simulink model "SistemaGrua_ModeloPlanta"  (R2020b)
settings: Solver=VariableStepAuto  StartTime=0.0  StopTime=10  RelTol=1e-3
values from neighbouring files (symbols this model uses):
  bhb = 1e8    (= 100000000)    [Valores.m]    (also in Valores_1.m; valoresPlanta.m; valoresPlanta_29_9_24.m; valoresPlanta_V3.m)
  bhEb = 2.2e9    (= 2200000000)    [Valores.m]    (also in Valores_1.m; valoresPlanta.m; valoresPlanta_29_9_24.m; valoresPlanta_V3.m)
  bhm = 18    [Valores.m]    (also in Valores_1.m; valoresPlanta.m; valoresPlanta_29_9_24.m; valoresPlanta_V3.m)
  bwu = 150    [Valores.m]    (also in Valores_1.m; valoresPlanta.m; valoresPlanta_29_9_24.m; valoresPlanta_V3.m)
  ih = 22    [Valores.m]    (also in Valores_1.m; valoresPlanta.m; valoresPlanta_29_9_24.m; valoresPlanta_V3.m)
  it = 30    [Valores.m]    (also in Valores_1.m; valoresPlanta.m; valoresPlanta_29_9_24.m; valoresPlanta_V3.m)
  Jhm_hb = 30    [Valores.m]    (also in Valores_1.m; valoresPlanta.m; valoresPlanta_29_9_24.m; valoresPlanta_V3.m)
  kwu = 2.36e8    (= 236000000)    [Valores.m]    (also in Valores_1.m; valoresPlanta.m; valoresPlanta_29_9_24.m; valoresPlanta_V3.m)
  rhd = 0.75    [Valores.m]    (also in Valores_1.m; valoresPlanta.m; valoresPlanta_29_9_24.m; valoresPlanta_V3.m)
  rtd = 0.5    [Valores.m]    (also in Valores_1.m; valoresPlanta.m; valoresPlanta_29_9_24.m; valoresPlanta_V3.m)
  tauhm = 1e-3    (= 0.001)    [Valores.m]    (also in Valores_1.m)
  Thb_Max = 5e4    (= 50000)    [Valores.m]    (also in Valores_1.m; valoresPlanta.m; valoresPlanta_29_9_24.m; valoresPlanta_V3.m)
  ThEb_Max = 1.1e6    (= 1100000)    [Valores.m]    (also in Valores_1.m; valoresPlanta.m; valoresPlanta_29_9_24.m; valoresPlanta_V3.m)
  Yt0 = 45    [Valores.m]    (also in Valores_1.m; valoresPlanta.m; valoresPlanta_29_9_24.m; valoresPlanta_V3.m)
undefined symbols (not defined in the file or in its folder): beqc, Meqc, sigbuilder_block
settings Model: Creator=Matias  LastModifiedBy=agustin

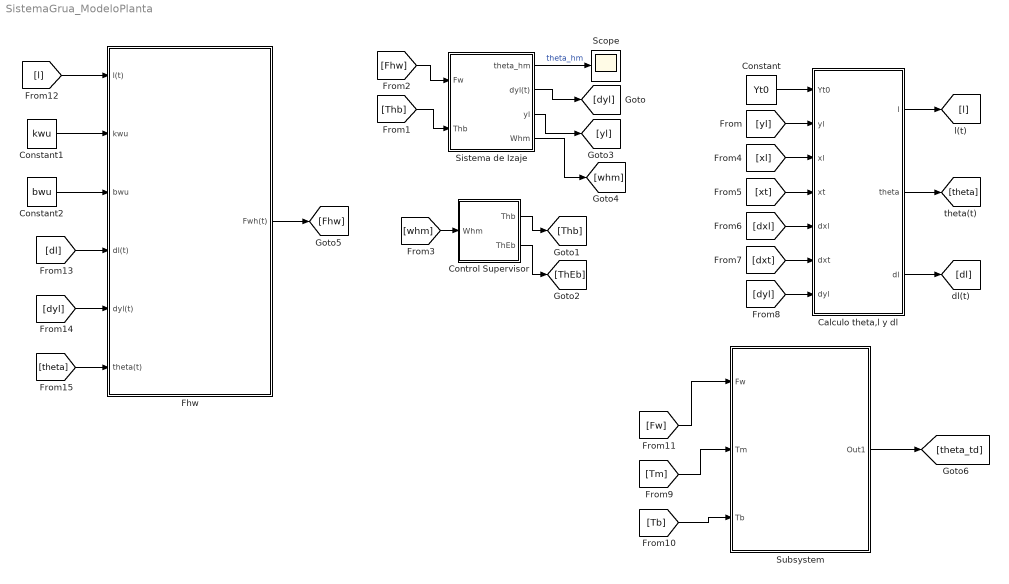
== system SistemaGrua_ModeloPlanta ==
  Calculo theta,l y dl : Subsystem
  Constant : Constant  Value=Yt0
  Constant1 : Constant  Value=kwu
  Constant2 : Constant  Value=bwu
  Control Supervisor : Subsystem
  Fhw : Subsystem
  Scope : Scope
  Sistema de Izaje : Subsystem
  Subsystem : Subsystem
  wires:
  [whm] -> Control Supervisor/1(Whm)
  Control Supervisor/1(Thb) -> [Thb]
  Sistema de Izaje/2(dyl(t)) -> [dyl]
  [Thb] -> Sistema de Izaje/2(Thb)
  [Fhw] -> Sistema de Izaje/1(Fw)
  Control Supervisor/2(ThEb) -> [ThEb]
  Sistema de Izaje/1(theta_hm) -> Scope/1  "theta_hm"
  Calculo theta,l y dl/1(l) -> [l]
  Calculo theta,l y dl/2(theta) -> [theta]
  Constant/1 -> Calculo theta,l y dl/1(Yt0)
  [xt] -> Calculo theta,l y dl/4(xt)
  [xl] -> Calculo theta,l y dl/3(xl)
  [yl] -> Calculo theta,l y dl/2(yl)
  Calculo theta,l y dl/3(dl) -> [dl]
  [dyl] -> Calculo theta,l y dl/7(dyl)
  [dxt] -> Calculo theta,l y dl/6(dxt)
  [dxl] -> Calculo theta,l y dl/5(dxl)
  Fhw/1(Fwh(t)) -> [Fhw]
  [theta] -> Fhw/6(theta(t))
  [dyl] -> Fhw/5(dyl(t))
  [dl] -> Fhw/4(dl(t))
  [l] -> Fhw/1(l(t))
  Constant1/1 -> Fhw/2(kwu)
  Constant2/1 -> Fhw/3(bwu)
  Sistema de Izaje/3(yl) -> [yl]
  Sistema de Izaje/4(Whm) -> [whm]
  [Tb] -> Subsystem/3(Tb)
  [Fw] -> Subsystem/1(Fw)
  [Tm] -> Subsystem/2(Tm)
  Subsystem/1(Out1) -> [theta_td]

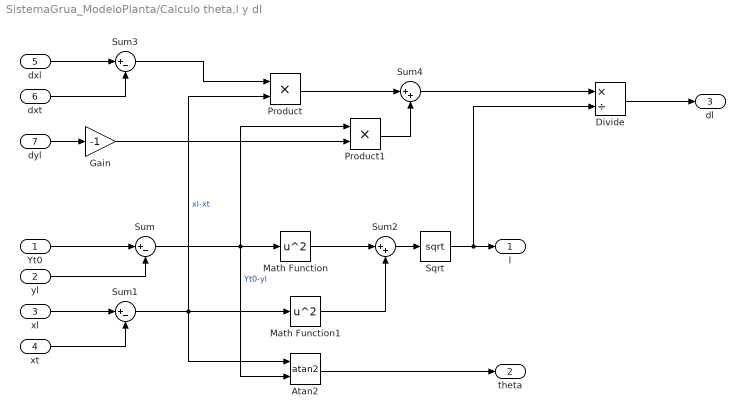
== system SistemaGrua_ModeloPlanta/Calculo theta,l y dl ==
  Yt0 : Inport
  yl : Inport  Port=2
  xl : Inport  Port=3
  xt : Inport  Port=4
  dxl : Inport  Port=5
  dxt : Inport  Port=6
  dyl : Inport  Port=7
  Atan2 : Trigonometry  Operator=atan2
  Divide : Product  Inputs=*/
  Gain : Gain  Gain=-1
  Math Function : Math  Operator=square  SaturateOnIntegerOverflow=on
  Math Function1 : Math  Operator=square  SaturateOnIntegerOverflow=on
  Product : Product
  Product1 : Product
  Sqrt : Sqrt  SaturateOnIntegerOverflow=on
  Sum : Sum  Inputs=|+-
  Sum1 : Sum  Inputs=|+-
  Sum2 : Sum  Inputs=|++
  Sum3 : Sum  Inputs=|+-
  Sum4 : Sum  Inputs=|++
  l : Outport
  theta : Outport  Port=2
  dl : Outport  Port=3
  wires:
  Yt0/1 -> Sum/1
  yl/1 -> Sum/2
  xl/1 -> Sum1/1
  xt/1 -> Sum1/2
  Atan2/1 -> theta/1
  Sum1/1 -> Product/2, Math Function1/1, Atan2/1  "xl-xt"
  Sum/1 -> Product1/1, Atan2/2, Math Function/1  "Yt0-yl"
  Math Function/1 -> Sum2/1
  Math Function1/1 -> Sum2/2
  Sum2/1 -> Sqrt/1
  Sqrt/1 -> Divide/2, l/1
  dxl/1 -> Sum3/1
  dxt/1 -> Sum3/2
  Sum3/1 -> Product/1
  dyl/1 -> Gain/1
  Gain/1 -> Product1/2
  Product/1 -> Sum4/1
  Product1/1 -> Sum4/2
  Sum4/1 -> Divide/1
  Divide/1 -> dl/1

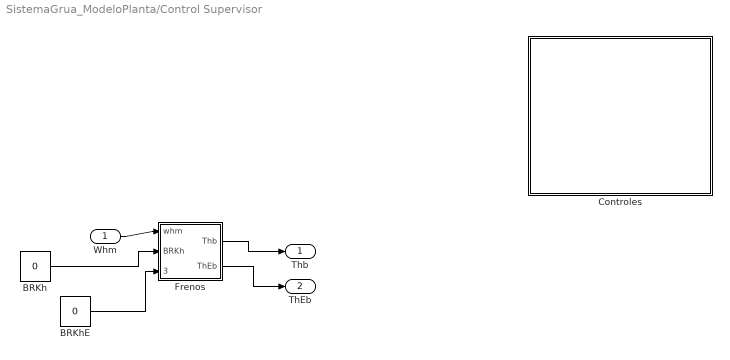
== system SistemaGrua_ModeloPlanta/Control Supervisor ==
  Whm : Inport
  BRKh : Constant  Value=0
  BRKhE : Constant  Value=0
  Controles : Subsystem
  "Frenos " : Stateflow chart  TreatAsAtomicUnit=on
  Thb : Outport
  ThEb : Outport  Port=2
  wires:
  "Frenos "/1(Thb) -> Thb/1
  BRKh/1 -> "Frenos "/2(BRKh)
  Whm/1 -> "Frenos "/1(whm)
  BRKhE/1 -> "Frenos "/3(BRKhE)
  "Frenos "/2(ThEb) -> ThEb/1

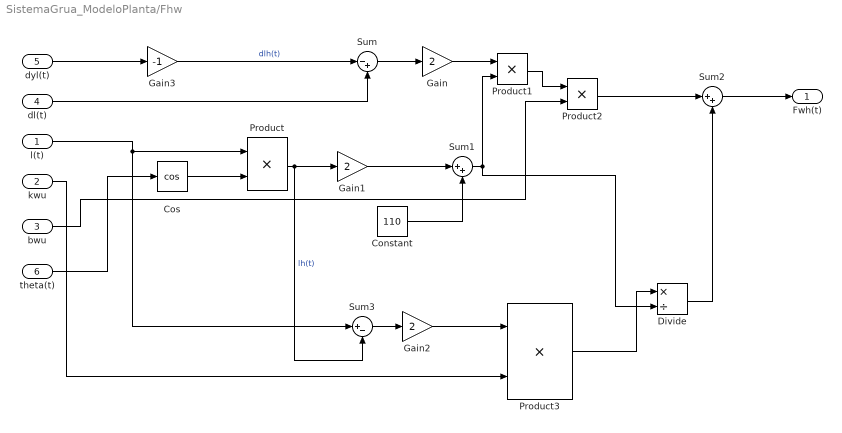
== system SistemaGrua_ModeloPlanta/Fhw ==
  l(t) : Inport
  kwu : Inport  Port=2
  bwu : Inport  Port=3
  dl(t) : Inport  Port=4
  dyl(t) : Inport  Port=5
  theta(t) : Inport  Port=6
  Constant : Constant  Value=110
  Cos : Trigonometry  Operator=cos
  Divide : Product  Inputs=*/
  Gain : Gain  Gain=2
  Gain1 : Gain  Gain=2
  Gain2 : Gain  Gain=2
  Gain3 : Gain  Gain=-1
  Product{,1..3} (4 alike) : Product
  Sum : Sum  Inputs=|-+
  Sum1 : Sum  Inputs=|++
  Sum2 : Sum  Inputs=|++
  Sum3 : Sum  Inputs=|+-
  Fwh(t) : Outport
  wires:
  dl(t)/1 -> Sum/2
  Sum/1 -> Gain/1
  Gain1/1 -> Sum1/1
  Product/1 -> Sum3/2, Gain1/1  "lh(t)"
  l(t)/1 -> Sum3/1, Product/1
  theta(t)/1 -> Cos/1
  Cos/1 -> Product/2
  Constant/1 -> Sum1/2
  Gain/1 -> Product1/1
  Sum1/1 -> Product1/2, Divide/2
  Product1/1 -> Product2/1
  bwu/1 -> Product2/2
  Product2/1 -> Sum2/1
  Sum3/1 -> Gain2/1
  Gain2/1 -> Product3/1
  kwu/1 -> Product3/2
  Product3/1 -> Divide/1
  Divide/1 -> Sum2/2
  Sum2/1 -> Fwh(t)/1
  dyl(t)/1 -> Gain3/1
  Gain3/1 -> Sum/1  "dlh(t)"

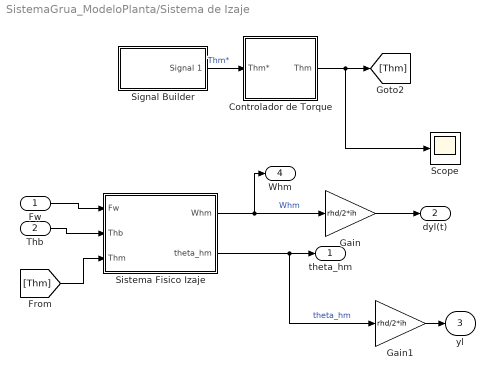
== system SistemaGrua_ModeloPlanta/Sistema de Izaje ==
  Fw : Inport
  Thb : Inport  Port=2
  Controlador de Torque : Subsystem
  Gain : Gain  Gain=rhd/2*ih
  Gain1 : Gain  Gain=rhd/2*ih
  Scope : Scope
  Signal Builder : Subsystem  Tag=STV Subsys  LoadFcn=sigbuilder_block('load');  StartFcn=sigbuilder_block('start');  StopFcn=sigbuilder_block('stop');  ClipboardFcn=sigbuilder_block('clipboard');  mask(Sigbuilder block){tuvar=[0:10]}
      mask help: Simulink:masks:SigbuilderBlock_MD
      mask init:
      | if ~strcmp(get_param(bdroot(gcbh),'SimulationStatus'),'stopped') tuvar = sigbuilder_block('maskInit'); end
      settings: CopyFcn=sigbuilder_block('copy');  DeleteFcn=sigbuilder_block('delete');  ModelCloseFcn=sigbuilder_block('modelClose');  PreSaveFcn=sigbuilder_block('preSave');  PauseFcn=sigbuilder_block('pause');  ContinueFcn=sigbuilder_block('continue');  NameChangeFcn=sigbuilder_block('namechange');  OpenFcn=sigbuilder_block('open',[5.4 36 1141.2 516.6 ]);  CloseFcn=sigbuilder_block('close');
      mask Display: plot(0, 0, 100, 100,[2, 2, 32, 32, 2], [68, 8, 8, 68, 68],[32, 2], [38, 38], [32, 19, 2],[53, 60, 44], [32, 17, 17, 2],[16, 16, 31, 31]);txt = getActiveGroup(gcbh);text(2, 100, txt,'verticalAlignment', 'top');
  Sistema Fisico Izaje : Subsystem
  theta_hm : Outport
  dyl(t) : Outport  Port=2
  yl : Outport  Port=3
  Whm : Outport  Port=4
  wires:
  Signal Builder/1(Signal 1) -> Controlador de Torque/1(Thm*)  "Thm*"
  Controlador de Torque/1(Thm) -> Scope/1, [Thm]
  Fw/1 -> Sistema Fisico Izaje/1(Fw)
  Thb/1 -> Sistema Fisico Izaje/2(Thb)
  Sistema Fisico Izaje/1(Whm) -> Whm/1, Gain/1  "Whm"
  Sistema Fisico Izaje/2(theta_hm) -> Gain1/1, theta_hm/1  "theta_hm"
  [Thm] -> Sistema Fisico Izaje/3(Thm)
  Gain/1 -> dyl(t)/1
  Gain1/1 -> yl/1

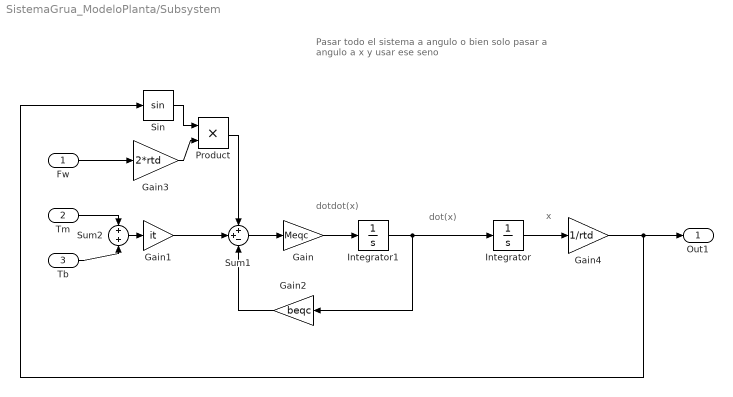
== system SistemaGrua_ModeloPlanta/Subsystem ==
  note: x
  note: dot(x)
  note: dotdot(x)
  note: Pasar todo el sistema a angulo
      | o bien solo pasar a angulo a x y usar ese seno
  Fw : Inport
  Tm : Inport  Port=2
  Tb : Inport  Port=3
  Gain : Gain  Gain=Meqc
  Gain1 : Gain  Gain=it
  Gain2 : Gain  Gain=beqc
  Gain3 : Gain  Gain=2*rtd
  Gain4 : Gain  Gain=1/rtd
  Integrator : Integrator
  Integrator1 : Integrator
  Product : Product
  Sin : Trigonometry
  Sum1 : Sum  Inputs=++-
  Sum2 : Sum
  Out1 : Outport
  wires:
  Sin/1 -> Product/1
  Gain1/1 -> Sum1/2
  Integrator1/1 -> Gain2/1, Integrator/1
  Sum2/1 -> Gain1/1
  Integrator/1 -> Gain4/1
  Gain3/1 -> Product/2
  Gain2/1 -> Sum1/3
  Gain/1 -> Integrator1/1
  Gain4/1 -> Sin/1, Out1/1
  Sum1/1 -> Gain/1
  Product/1 -> Sum1/1
  Fw/1 -> Gain3/1
  Tb/1 -> Sum2/2
  Tm/1 -> Sum2/1

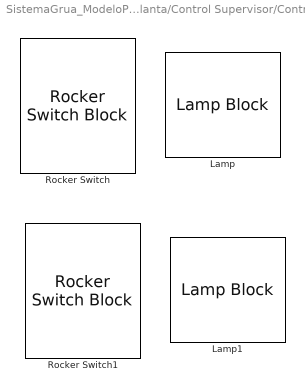
== system SistemaGrua_ModeloPlanta/Control Supervisor/Controles ==
  Lamp : LampBlock
  Lamp1 : LampBlock
  Rocker Switch : RockerSwitchBlock
      settings: Values={{'Off', 'On'}, [0 1]}
  Rocker Switch1 : RockerSwitchBlock
      settings: Values={{'Off', 'On'}, [0 1]}

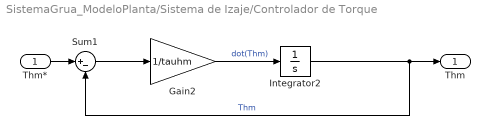
== system SistemaGrua_ModeloPlanta/Sistema de Izaje/Controlador de Torque ==
  Thm* : Inport
  Gain2 : Gain  Gain=1/tauhm
  Integrator2 : Integrator
  Sum1 : Sum  Inputs=|+-
  Thm : Outport
  wires:
  Integrator2/1 -> Thm/1, Sum1/2  "Thm"
  Thm*/1 -> Sum1/1
  Sum1/1 -> Gain2/1
  Gain2/1 -> Integrator2/1  "dot(Thm)"

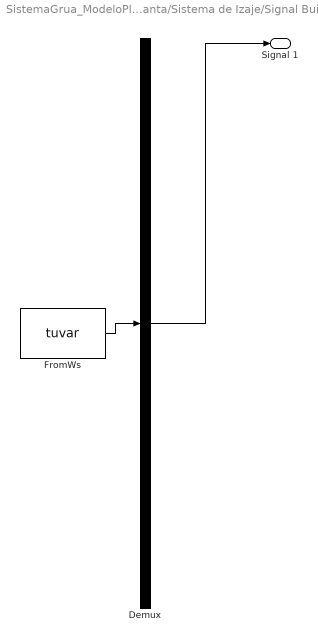
== system SistemaGrua_ModeloPlanta/Sistema de Izaje/Signal Builder ==
  Demux : Demux  Tag=STV Demux  Outputs=1
      settings: DisplayOption=none
  FromWs : FromWorkspace  Tag=STV FromWs  VariableName=tuvar
      SigBuilderData=|
      | common.afterFinalStr = 'Extrapolate'
      | common.sampleTime = 0
      | dataSet.timeRange = [0 10]
      | dataSet.name = 'Group 1'
      | sbobj.Groups.Name = 'Group 1'
      | sbobj.Groups.Signals.Name = 'Signal 1'
      | sbobj.Groups.Signals.XData = [0 4 6 10]
      | sbobj.Groups.Signals.YData = [0 20000 20000 0]
  Signal 1 : Outport  Tag=STV Outport
  wires:
  Demux/1 -> Signal 1/1
  FromWs/1 -> Demux/1

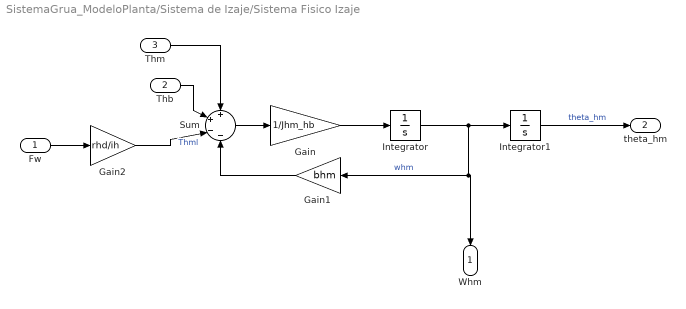
== system SistemaGrua_ModeloPlanta/Sistema de Izaje/Sistema Fisico Izaje ==
  Fw : Inport
  Thb : Inport  Port=2
  Thm : Inport  Port=3
  Gain : Gain  Gain=1/Jhm_hb
  Gain1 : Gain  Gain=bhm
  Gain2 : Gain  Gain=rhd/ih
  Integrator : Integrator
  Integrator1 : Integrator
  Sum : Sum  Inputs=++--
  Whm : Outport
  theta_hm : Outport  Port=2
  wires:
  Gain/1 -> Integrator/1
  Sum/1 -> Gain/1
  Integrator/1 -> Whm/1, Gain1/1, Integrator1/1  "whm"
  Fw/1 -> Gain2/1
  Gain1/1 -> Sum/4
  Thb/1 -> Sum/2
  Thm/1 -> Sum/1
  Integrator1/1 -> theta_hm/1  "theta_hm"
  Gain2/1 -> Sum/3  "Thml"

== stateflow chart SistemaGrua_ModeloPlanta/Control Supervisor/Frenos  ==
  state FrenosOperacion
    state BRKh_off
      during:
      Thb=-bhb*whm;
      Thb=min(Thb_Max,Thb);
    state BRKh_on
      during:
      Thb=0;
    (default) -> BRKh_off
    BRKh_off -> BRKh_on [order 1] : [BRKh==1 && BRKhE==1]
    BRKh_on -> BRKh_off [order 1] : [BRKh==0 && BRKhE==1]
  state FrenosEmergencia
    state BRKhE_off
      during:
      ThEb=-bhEb*whm;
      ThEb=min(ThEb_Max,ThEb);
    state BRKhE_on
      during:
      ThEb=0;
    (default) -> BRKhE_off
    BRKhE_off -> BRKhE_on : [BRKhE==1]
    BRKhE_on -> BRKhE_off [order 1] : [BRKhE==0]
  BRKh_on -> FrenosEmergencia [order 2] : [BRKhE==0]
  BRKh_off -> FrenosEmergencia [order 2] : [BRKhE==0]
  BRKhE_on -> FrenosOperacion [order 2] : [BRKhE==1]
  (default) -> FrenosEmergencia
  data: Thb output; whm input; bhb parameter; Thb_Max parameter; BRKh input; ThEb output; bhEb parameter; ThEb_Max parameter; BRKhE input
